simulink library "constX_YZvarT_ADCPTurb_cl"  (R2018b)
settings: Solver=VariableStepAuto  StartTime=0.0  StopTime=10.0  RelTol=1e-3
undefined symbols (not defined in the file): env
libraries: variableFlowProfileCalculationYZ_ul x1
settings Model: Creator=jcreed2  LastModifiedBy=jcreed2

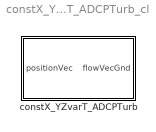
== system constX_YZvarT_ADCPTurb_cl ==
  constX_YZvarT_ADCPTurb : Subsystem

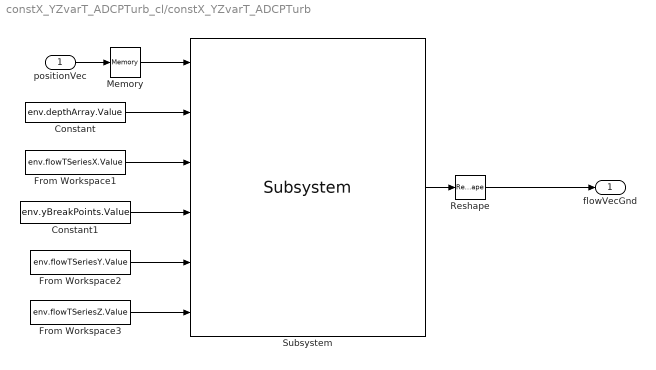
== system constX_YZvarT_ADCPTurb_cl/constX_YZvarT_ADCPTurb ==
  positionVec : Inport
  Constant : Constant  Value=env.depthArray.Value
  Constant1 : Constant  Value=env.yBreakPoints.Value
  From Workspace1 : FromWorkspace  VariableName=env.flowTSeriesX.Value  SampleTime=0
  From Workspace2 : FromWorkspace  VariableName=env.flowTSeriesY.Value  SampleTime=0
  From Workspace3 : FromWorkspace  VariableName=env.flowTSeriesZ.Value  SampleTime=0
  Memory : Memory
  Reshape : Reshape  OutputDimensionality=Column vector (2-D)
  Subsystem : variableFlowProfileCalculationYZ_ul/variableFlowProfileCalculation/Subsystem  SystemSampleTime=-1
  flowVecGnd : Outport
  wires:
  Constant/1 -> Subsystem/2
  positionVec/1 -> Memory/1
  Memory/1 -> Subsystem/1
  Reshape/1 -> flowVecGnd/1
  From Workspace1/1 -> Subsystem/3
  Subsystem/1 -> Reshape/1
  Constant1/1 -> Subsystem/4
  From Workspace3/1 -> Subsystem/6
  From Workspace2/1 -> Subsystem/5
